simulink model "ball_on_beam_sim_HW_10"  (R2018a)
settings: Solver=ode45  StartTime=0.0  StopTime=100  MaxStep=1  RelTol=1e-3
InitFcn:
  | ball_on_beam_param
undefined symbols (not defined in the file or in its folder): ball_on_beam_animation, ball_on_beam_ctrl, Par
settings Model: Creator=canla  LastModifiedBy=canla
settings OptimizationCC: LifeSpan=inf

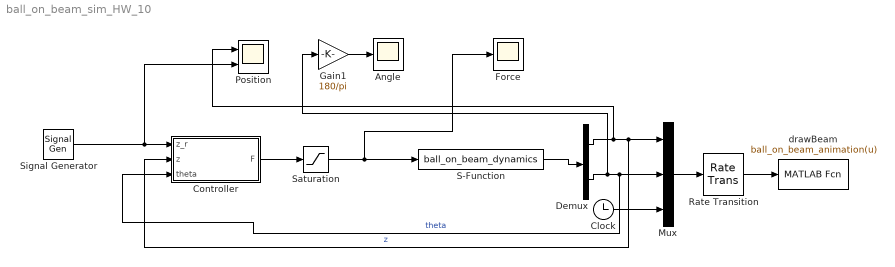
== system ball_on_beam_sim_HW_10 ==
  Angle : Scope
  Clock : Clock
  Controller : Subsystem
  Demux : Demux  Outputs=2
  Force : Scope
  Gain1 : Gain  Gain=180/pi
  Mux : Mux  Inputs=3
  Position : Scope  NumInputPorts=2
  Rate Transition : RateTransition  OutPortSampleTime=Par.t_plot
  S-Function : S-Function  FunctionName=ball_on_beam_dynamics  Parameters=Par  SFunctionDeploymentMode=off  EnableBusSupport=off
  Saturation : Saturate  UpperLimit=Par.F_max  LowerLimit=-Par.F_max
  Signal Generator : SignalGenerator  WaveForm=square  Amplitude=0.5  Frequency=0.05
  drawBeam : MATLABFcn  MATLABFcn=ball_on_beam_animation(u)  OutputDimensions=0
  wires:
  S-Function/1 -> Demux/1
  Demux/2 -> Gain1/1, Controller/3(theta), Mux/2  "theta"
  Demux/1 -> Position/1, Controller/2(z), Mux/1  "z"
  Clock/1 -> Mux/3
  Mux/1 -> Rate Transition/1
  Rate Transition/1 -> drawBeam/1
  Gain1/1 -> Angle/1
  Signal Generator/1 -> Position/2, Controller/1(z_r)
  Controller/1(F) -> Saturation/1
  Saturation/1 -> S-Function/1, Force/1

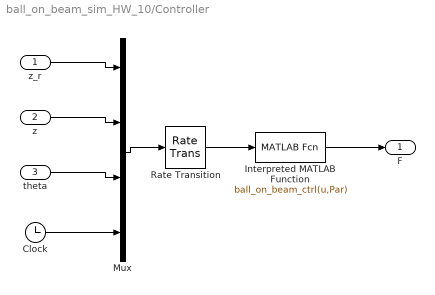
== system ball_on_beam_sim_HW_10/Controller ==
  z_r : Inport
  z : Inport  Port=2
  theta : Inport  Port=3
  Clock : Clock
  Interpreted MATLAB Function : MATLABFcn  MATLABFcn=ball_on_beam_ctrl(u,Par)
  Mux : Mux
  Rate Transition : RateTransition  OutPortSampleTime=Par.Ts
  F : Outport
  wires:
  z_r/1 -> Mux/1
  z/1 -> Mux/2
  theta/1 -> Mux/3
  Mux/1 -> Rate Transition/1
  Rate Transition/1 -> Interpreted MATLAB Function/1
  Interpreted MATLAB Function/1 -> F/1
  Clock/1 -> Mux/4
